simulink model "Bat_Dinamic_v10"  (R2022b)
settings: Solver=ode23t  StartTime=0.0  StopTime=81000  FixedStep=1  RelTol=1e-3
values from neighbouring files (symbols this model uses):
  Ec0 = 20.142    [Initializer.m]
  Ec10 = 0.012506    [Initializer.m]
  Ed0 = 24.129    [Initializer.m]
  Ed10 = -0.012749    [Initializer.m]
  Phi0 = 374.5    [Initializer.m]
  R1 = 0.016495    [Initializer.m]
  R2 = 0.00014539    [Initializer.m]
  Rc = 0.26    [Initializer.m]
  Rd = 0.0171277    [Initializer.m]
  V0 = 24    [Initializer.m]
undefined symbols (not defined in the file or in its folder): magnitude
libraries: fl_lib x13, nesl_utility x5
settings Model: Creator=Alberto  LastModifiedBy=judow
settings SolverCC: AlgebraicLoopSolver=TrustRegion
settings DebuggingCC: UnconnectedInputMsg=warning  UnconnectedOutputMsg=warning  UnconnectedLineMsg=warning  SFMachineParentedDataDiag=warning
settings ModelReferenceCC: EnableRefExpFcnMdlSchedulingChecks=on

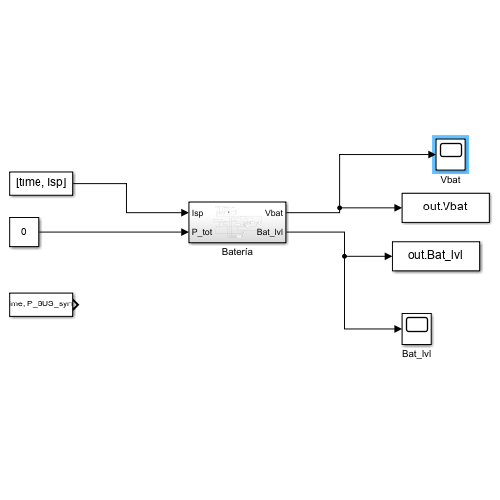
[thumbnail: Simulink's stored preview of the top-level diagram]
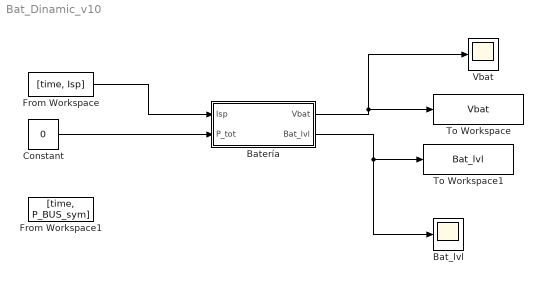
== system Bat_Dinamic_v10 ==
  Bat_lvl : Scope
  Batería : Subsystem
  Constant : Constant  Value=0
  From Workspace : FromWorkspace  VariableName=[time, Isp]
  From Workspace1 : FromWorkspace  VariableName=[time, P_BUS_sym]
  To Workspace : ToWorkspace  VariableName=Vbat  SaveFormat=Timeseries  SampleTime=-1
  To Workspace1 : ToWorkspace  VariableName=Bat_lvl  SaveFormat=Timeseries  SampleTime=-1
  Vbat : Scope
  wires:
  From Workspace/1 -> Batería/1(Isp)
  Batería/1(Vbat) -> To Workspace/1, Vbat/1
  Batería/2(Bat_lvl) -> To Workspace1/1, Bat_lvl/1
  Constant/1 -> Batería/2(P_tot)

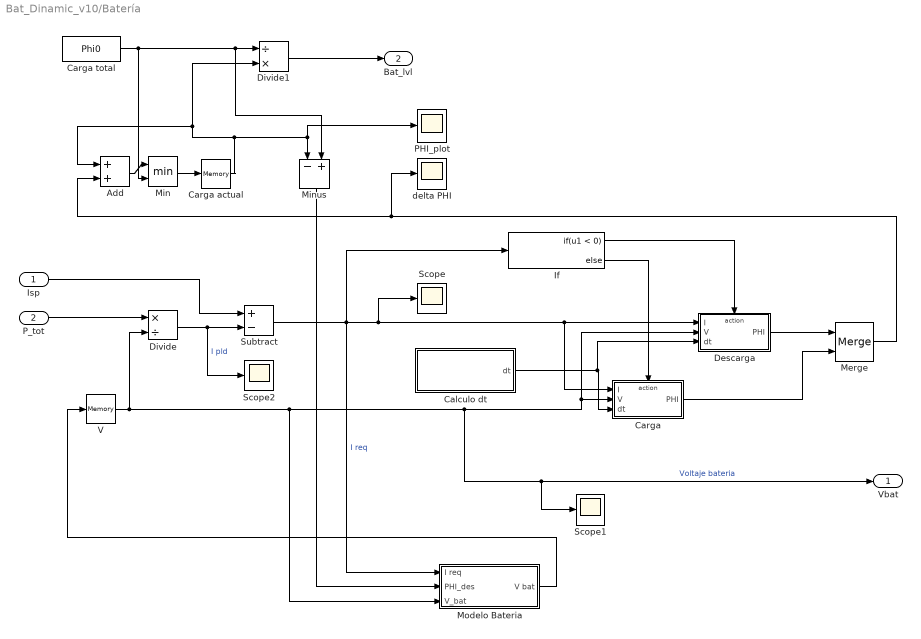
== system Bat_Dinamic_v10/Batería ==
  Isp : Inport
  P_tot : Inport  Port=2
  Add : Sum
  Calculo dt : Subsystem
  Carga : Subsystem  TreatAsAtomicUnit=on
  Carga actual : Memory  InheritSampleTime=on
  Carga total : Constant  Value=Phi0
  Descarga : Subsystem  TreatAsAtomicUnit=on
  Divide : Product  Inputs=*/
  Divide1 : Product  Inputs=/*
  If : If  IfExpression=u1 < 0
  Merge : Merge
  Min : MinMax  Inputs=2  ZeroCross=off
  Minus : Sum  Inputs=-+
  Modelo Bateria : Subsystem
  PHI_plot : Scope
  Scope : Scope
  Scope1 : Scope
  Scope2 : Scope
  Subtract : Sum  Inputs=+-
  V : Memory  InitialCondition=V0
  delta PHI : Scope
  Vbat : Outport
  Bat_lvl : Outport  Port=2
  wires:
  Merge/1 -> Add/2, delta PHI/1
  Modelo Bateria/1(V bat) -> V/1
  Carga total/1 -> Min/2, Minus/2, Divide1/1
  Divide1/1 -> Bat_lvl/1
  Descarga/1(PHI) -> Merge/1
  Carga/1(PHI) -> Merge/2
  Carga actual/1 -> Add/1, Divide1/2, PHI_plot/1, Minus/1
  If/2 -> Carga/Action
  If/1 -> Descarga/Action
  Subtract/1 -> If/1, Modelo Bateria/1(I req), Scope/1, Carga/1(I), Descarga/1(I)  "I req"
  P_tot/1 -> Divide/1
  V/1 -> Divide/2, Scope1/1, Vbat/1, Descarga/2(V), Carga/2(V), Modelo Bateria/3(V_bat)  "Voltaje bateria"
  Divide/1 -> Scope2/1, Subtract/2  "I pld"
  Isp/1 -> Subtract/1
  Minus/1 -> Modelo Bateria/2(PHI_des)
  Calculo dt/1(dt) -> Descarga/3(dt), Carga/3(dt)
  Add/1 -> Min/1
  Min/1 -> Carga actual/1

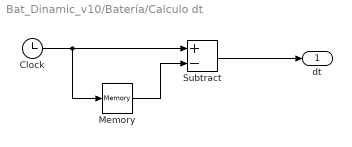
== system Bat_Dinamic_v10/Batería/Calculo dt ==
  Clock : Clock
  Memory : Memory
  Subtract : Sum  Inputs=+-
  dt : Outport
  wires:
  Clock/1 -> Memory/1, Subtract/1
  Subtract/1 -> dt/1
  Memory/1 -> Subtract/2

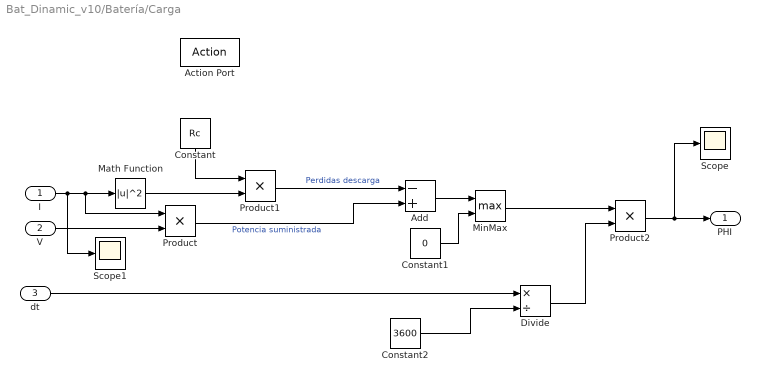
== system Bat_Dinamic_v10/Batería/Carga ==
  I : Inport
  V : Inport  Port=2
  dt : Inport  Port=3
  Action Port : ActionPort  ActionPortLabel=else
  Add : Sum  Inputs=-+
  Constant : Constant  Value=Rc
  Constant1 : Constant  Value=0
  Constant2 : Constant  Value=3600
  Divide : Product  Inputs=*/
  Math Function : Math  Operator=magnitude^2
  MinMax : MinMax  Function=max  Inputs=2
  Product : Product
  Product1 : Product
  Product2 : Product
  Scope : Scope
  Scope1 : Scope
  PHI : Outport
  wires:
  I/1 -> Scope1/1, Product/1, Math Function/1
  Product1/1 -> Add/1  "Perdidas descarga"
  Math Function/1 -> Product1/2
  Constant/1 -> Product1/1
  V/1 -> Product/2
  Product/1 -> Add/2  "Potencia suministrada"
  Add/1 -> MinMax/1
  Constant1/1 -> MinMax/2
  MinMax/1 -> Product2/1
  Product2/1 -> Scope/1, PHI/1
  Divide/1 -> Product2/2
  dt/1 -> Divide/1
  Constant2/1 -> Divide/2

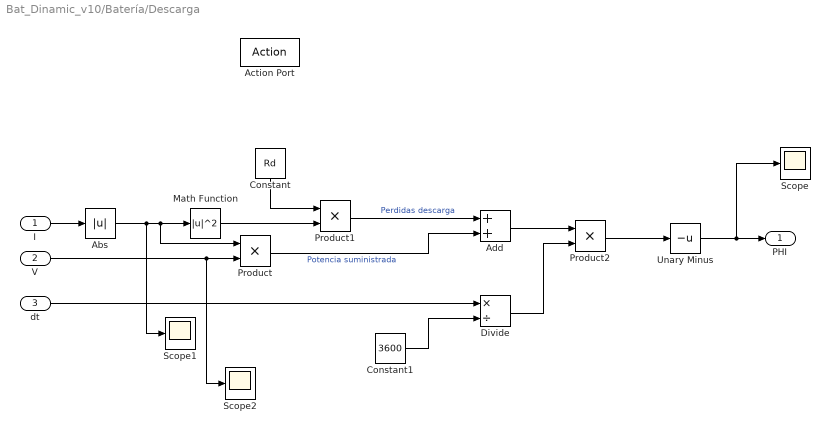
== system Bat_Dinamic_v10/Batería/Descarga ==
  I : Inport
  V : Inport  Port=2
  dt : Inport  Port=3
  Action Port : ActionPort  ActionPortLabel=if(u1 < 0)
  Abs : Abs  SaturateOnIntegerOverflow=off
  Add : Sum
  Constant : Constant  Value=Rd
  Constant1 : Constant  Value=3600
  Divide : Product  Inputs=*/
  Math Function : Math  Operator=magnitude^2
  Product : Product
  Product1 : Product
  Product2 : Product
  Scope : Scope
  Scope1 : Scope
  Scope2 : Scope
  Unary Minus : UnaryMinus
  PHI : Outport
  wires:
  Math Function/1 -> Product1/2
  Product/1 -> Add/2  "Potencia suministrada"
  Constant/1 -> Product1/1
  Product1/1 -> Add/1  "Perdidas descarga"
  I/1 -> Abs/1
  V/1 -> Scope2/1, Product/2
  Add/1 -> Product2/1
  Product2/1 -> Unary Minus/1
  Divide/1 -> Product2/2
  Abs/1 -> Scope1/1, Product/1, Math Function/1
  Unary Minus/1 -> Scope/1, PHI/1
  dt/1 -> Divide/1
  Constant1/1 -> Divide/2

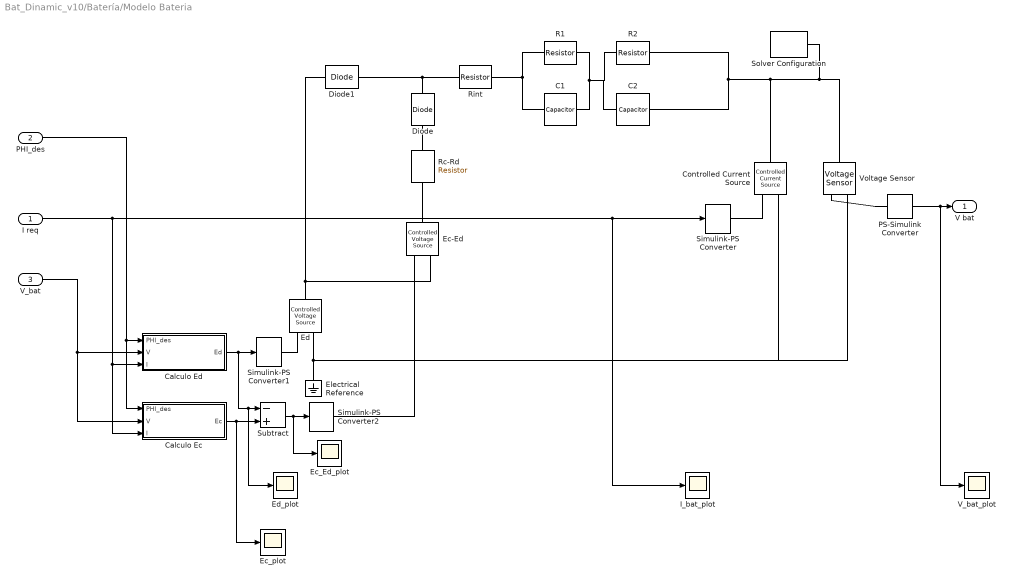
== system Bat_Dinamic_v10/Batería/Modelo Bateria ==
  I req : Inport
  PHI_des : Inport  Port=2
  V_bat : Inport  Port=3
  C1 : fl_lib/Electrical/Electrical Elements/Capacitor  c=C1 F  r=1e-12 Ohm  g=1e-12 1/Ohm  i_specify=off  i_priority=High  i=0 A  i_nominal_specify=off  i_nominal_unit=A  i_nominal_value=1  v_specify=off  v_priority=High  v=0 V  v_nominal_specify=off  v_nominal_unit=V  v_nominal_value=1  vc_specify=off  vc_priority=High  vc=0 V  vc_nominal_specify=off  vc_nominal_unit=V  vc_nominal_value=1
  C2 : fl_lib/Electrical/Electrical Elements/Capacitor  c=C2 F  r=1e-12 Ohm  g=1e-12 1/Ohm  i_specify=off  i_priority=High  i=0 A  i_nominal_specify=off  i_nominal_unit=A  i_nominal_value=1  v_specify=off  v_priority=High  v=0 V  v_nominal_specify=off  v_nominal_unit=V  v_nominal_value=1  vc_specify=off  vc_priority=High  vc=0 V  vc_nominal_specify=off  vc_nominal_unit=V  vc_nominal_value=1
  Calculo Ec : Subsystem
  Calculo Ed : Subsystem
  Controlled Current Source : fl_lib/Electrical/Electrical Sources/Controlled Current Source
  Diode : fl_lib/Electrical/Electrical Elements/Diode  Vf=1e-12 V  Ron=1e-12 Ohm  Goff=1e-12 1/Ohm  i_specify=off  i_priority=None  i=0 A  i_nominal_specify=off  i_nominal_unit=A  i_nominal_value=1  v_specify=off  v_priority=None  v=0 V  v_nominal_specify=off  v_nominal_unit=V  v_nominal_value=1
  Diode1 : fl_lib/Electrical/Electrical Elements/Diode  Vf=1e-12 V  Ron=1e-12 Ohm  Goff=1e-12 1/Ohm  i_specify=off  i_priority=None  i=0 A  i_nominal_specify=off  i_nominal_unit=A  i_nominal_value=1  v_specify=off  v_priority=None  v=0 V  v_nominal_specify=off  v_nominal_unit=V  v_nominal_value=1
  Ec-Ed : fl_lib/Electrical/Electrical Sources/Controlled Voltage Source
  Ec_Ed_plot : Scope
  Ec_plot : Scope
  Ed : fl_lib/Electrical/Electrical Sources/Controlled Voltage Source
  Ed_plot : Scope
  Electrical Reference : fl_lib/Electrical/Electrical Elements/Electrical Reference
  I_bat_plot : Scope
  PS-Simulink Converter : nesl_utility/PS-Simulink Converter  PhysicalDomain=network_engine_domain  SubClassName=ps_output  LeftPortType=input  RightPortType=output  PseudoPeriodic=off  Frequencies=[]  VectorFormat=1-D array  Unit=V  AffineConversion=off
  R1 : fl_lib/Electrical/Electrical Elements/Resistor  R=R1 Ohm  i_specify=off  i_priority=High  i=0 A  i_nominal_specify=off  i_nominal_unit=A  i_nominal_value=1  v_specify=off  v_priority=High  v=0 V  v_nominal_specify=off  v_nominal_unit=V  v_nominal_value=1
  R2 : fl_lib/Electrical/Electrical Elements/Resistor  R=R2 Ohm  i_specify=off  i_priority=High  i=0 A  i_nominal_specify=off  i_nominal_unit=A  i_nominal_value=1  v_specify=off  v_priority=High  v=0 V  v_nominal_specify=off  v_nominal_unit=V  v_nominal_value=1
  Rc-Rd : fl_lib/Electrical/Electrical Elements/Resistor  R=Rc-Rd Ohm  i_specify=off  i_priority=High  i=0 A  i_nominal_specify=off  i_nominal_unit=A  i_nominal_value=1  v_specify=off  v_priority=High  v=0 V  v_nominal_specify=off  v_nominal_unit=V  v_nominal_value=1
  Rint : fl_lib/Electrical/Electrical Elements/Resistor  R=Rd-R1-R2 Ohm  i_specify=off  i_priority=High  i=0 A  i_nominal_specify=off  i_nominal_unit=A  i_nominal_value=1  v_specify=off  v_priority=High  v=0 V  v_nominal_specify=off  v_nominal_unit=V  v_nominal_value=1
  Simulink-PS Converter : nesl_utility/Simulink-PS Converter  PhysicalDomain=network_engine_domain  SubClassName=ps_input  LeftPortType=input  RightPortType=output  PseudoPeriodic=off  Frequencies=[]  NoiseDistribution=none  NoiseParameters=[]  Unit=A  AffineConversion=off  FilteringAndDerivatives=zero  SimscapeFilterOrder=1  InputFilterTimeConstant=0.001  UdotUserProvided=1
  Simulink-PS Converter1 : nesl_utility/Simulink-PS Converter  PhysicalDomain=network_engine_domain  SubClassName=ps_input  LeftPortType=input  RightPortType=output  PseudoPeriodic=off  Frequencies=[]  NoiseDistribution=none  NoiseParameters=[]  Unit=V  AffineConversion=off  FilteringAndDerivatives=zero  SimscapeFilterOrder=1  InputFilterTimeConstant=0.001  UdotUserProvided=1
  Simulink-PS Converter2 : nesl_utility/Simulink-PS Converter  PhysicalDomain=network_engine_domain  SubClassName=ps_input  LeftPortType=input  RightPortType=output  PseudoPeriodic=off  Frequencies=[]  NoiseDistribution=none  NoiseParameters=[]  Unit=V  AffineConversion=off  FilteringAndDerivatives=zero  SimscapeFilterOrder=1  InputFilterTimeConstant=0.001  UdotUserProvided=1
  Solver Configuration : nesl_utility/Solver Configuration  PhysicalDomain=network_engine_domain  SubClassName=solver  LeftPortType=input  RightPortType=generic  Tones=[]  Harmonics=[]  SimulateNoise=off  Profile=off  UseLocalSampling=off  EnableSwitchedLinearOptims=on  FrequencyDomain=off  UseCCode=off  RelTol=0.001  AbsTol=1e-06  MinStep=1e-09  ToWorkspace=off  RevertToSquareIcSolve=off  NumHomotopyIterations=100  PhasorMode=off  PhasorModeNumHarmonics=1  ConsistencySolver=NEWTON_FTOL  IndexReductionMethod=DerivativeReplacement  DoDC=off  ResidualTolerance=1e-9  ConsistencyTolSource=GLOBAL  ConsistencyAbsTol=0.001  ConsistencyRelTol=0.001  ConsistencyTolFactor=0.001  UseLocalSolver=off  LocalSolverChoice=NE_BACKWARD_EULER_ADVANCER  ResolveIndetEquations=on  FunctionEvalNumThread=1  LocalSolverSampleTime=0.001  DoFixedCost=off  MaxNonlinIter=3  MaxModeIter=2  ComputeImpulses=off  ImpulseIterations=2  LinearAlgebra=Sparse  LinearAlgebraNumThread=0  EquationFormulation=NE_TIME_EF  DelaysMemoryBudget=1024  AutomaticFiltering=on  FilteringTimeConstant=0.001  PartitionStorageMethod=AS_NEEDED  PartitionMemoryBudget=1024  PartitionMethod=FAST
  Subtract : Sum  Inputs=-+
  V_bat_plot : Scope
  Voltage Sensor : fl_lib/Electrical/Electrical Sensors/Voltage Sensor
  V bat : Outport
  wires:
  Calculo Ec/1(Ec) -> Ec_plot/1, Subtract/2
  Calculo Ed/1(Ed) -> Ed_plot/1, Subtract/1, Simulink-PS Converter1/1
  Subtract/1 -> Ec_Ed_plot/1, Simulink-PS Converter2/1
  I req/1 -> Calculo Ec/3(I), Calculo Ed/3(I), I_bat_plot/1, Simulink-PS Converter/1
  PS-Simulink Converter/1 -> V_bat_plot/1, V bat/1
  PHI_des/1 -> Calculo Ec/1(PHI_des), Calculo Ed/1(PHI_des)
  V_bat/1 -> Calculo Ec/2(V), Calculo Ed/2(V)
  connections:
  R1/LConn1 -- C1/RConn1 -- Rint/LConn1
  Diode/LConn1 -- Rint/RConn1 -- Diode1/RConn1
  R1/RConn1 -- R2/LConn1 -- C2/RConn1 -- C1/LConn1
  Ec-Ed/RConn2 -- Ed/LConn1 -- Diode1/LConn1
  C2/LConn1 -- Solver Configuration/RConn1 -- Voltage Sensor/LConn1 -- Controlled Current Source/LConn1 -- R2/RConn1
  Ec-Ed/LConn1 -- Rc-Rd/LConn1
  Diode/RConn1 -- Rc-Rd/RConn1
  Simulink-PS Converter1/RConn1 -- Ed/RConn1
  Simulink-PS Converter2/RConn1 -- Ec-Ed/RConn1
  Electrical Reference/LConn1 -- Controlled Current Source/RConn2 -- Voltage Sensor/RConn2 -- Ed/RConn2
  Simulink-PS Converter/RConn1 -- Controlled Current Source/RConn1
  PS-Simulink Converter/LConn1 -- Voltage Sensor/RConn1

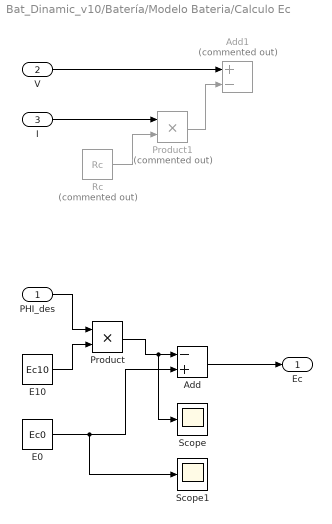
== system Bat_Dinamic_v10/Batería/Modelo Bateria/Calculo Ec ==
  PHI_des : Inport
  V : Inport  Port=2
  I : Inport  Port=3
  Add : Sum  Inputs=-+
  Add1 : Sum  Commented=on  Inputs=+-
  E0 : Constant  Value=Ec0
  E10 : Constant  Value=Ec10
  Product : Product
  Product1 : Product  Commented=on
  Rc : Constant  Commented=on  Value=Rc
  Scope : Scope
  Scope1 : Scope
  Ec : Outport
  wires:
  Product/1 -> Scope/1, Add/1
  E10/1 -> Product/2
  E0/1 -> Scope1/1, Add/2
  I/1 -> Product1/1
  Rc/1 -> Product1/2
  V/1 -> Add1/1
  Product1/1 -> Add1/2
  PHI_des/1 -> Product/1
  Add/1 -> Ec/1

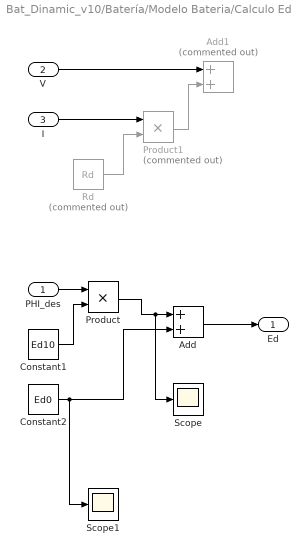
== system Bat_Dinamic_v10/Batería/Modelo Bateria/Calculo Ed ==
  PHI_des : Inport
  V : Inport  Port=2
  I : Inport  Port=3
  Add : Sum
  Add1 : Sum  Commented=on
  Constant1 : Constant  Value=Ed10
  Constant2 : Constant  Value=Ed0
  Product : Product
  Product1 : Product  Commented=on
  Rd : Constant  Commented=on  Value=Rd
  Scope : Scope
  Scope1 : Scope
  Ed : Outport
  wires:
  Product/1 -> Scope/1, Add/1
  Constant1/1 -> Product/2
  Constant2/1 -> Scope1/1, Add/2
  I/1 -> Product1/1
  Rd/1 -> Product1/2
  V/1 -> Add1/1
  Product1/1 -> Add1/2
  PHI_des/1 -> Product/1
  Add/1 -> Ed/1
